simulink model "sim_finale_1"  (R2024a)
settings: Solver=FixedStepAuto  StartTime=0.0  StopTime=40  FixedStep=0.001  RelTol=1e-3
undefined symbols (not defined in the file): A_p, A_y, aero_variabile_con_M, Attitude_0, Attitude_riferimento, b, B_p, B_pz, B_y, B_yz, C_A, C_l, C_m_alpha, C_N_alpha, C_p, C_y, conv_cost_distE, conv_cost_distN, conv_cost_eta, conv_cost_p, conv_cost_y, conv_cost_zeta, D_pz, D_yz, Env, F, G_wE, G_wN, G_xp, G_xy, I_sp, inertia_p, inertia_s, inertia_tot, L, m_p, m_s, m_tot, MIL, Moderate, P_p, P_y, R, r_cp_cm, r_nozzle_cm, S_rif, spinta_variabile, T_c, T_r, v_0, V_r, VelocitB_riferimento, w_0
libraries: cstblocks x16, simulink_extras x5, slpidlib x4, simulink x3, aerolibasang x3, aerolibwind2 x3, matrix_library x2, shared6dof x2, aerolibatmos2 x2, aerolibutil x1, aerolibanim x1
(part 1 of 2)
settings Model: Creator=leo  LastModifiedBy=seraf

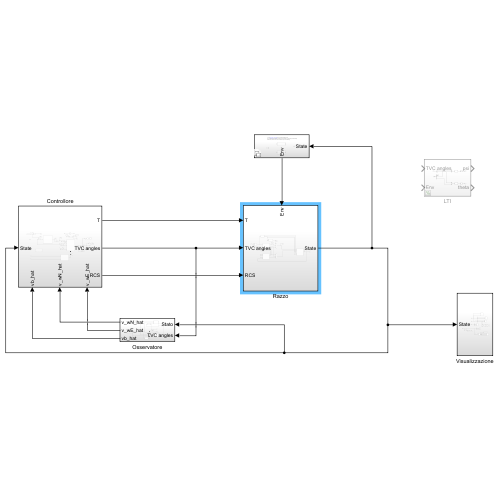
[thumbnail: Simulink's stored preview of the top-level diagram]
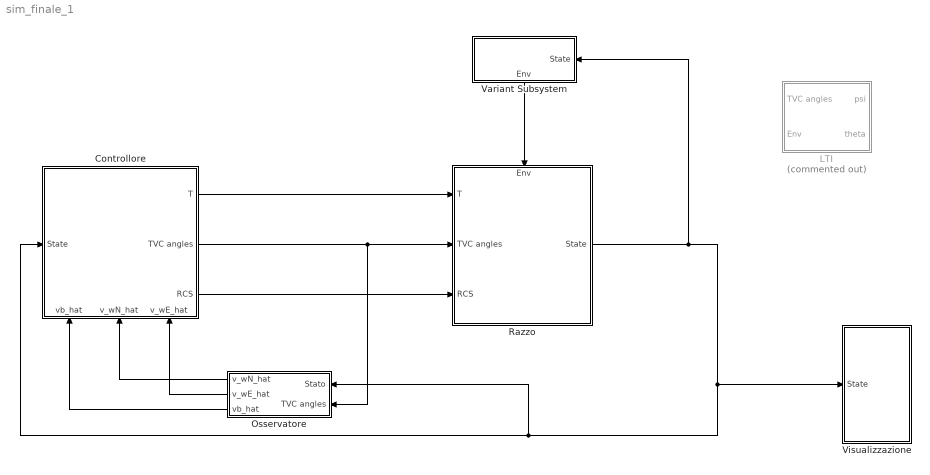
== system sim_finale_1 ==
  Controllore : Subsystem
      settings: PortSchema="{\"entries\":[{\"content\":{\"sides\":[{\"content\":{\"connectorIds\":[\"In1\"]},\"type\":\"ConnectorPlacement.EquallySpacedRectSide\",\"uuid\":\"b78b4143-dd7d-457a-9779-532a64936aad\"},{\"content\":{\"connectorIds\":[\"Out1\",\"Out2\",\"Out3\"],\"side\":\"RIGHT\"},\"type\":\"ConnectorPlacement.EquallySpacedRectSide\",\"uuid\":\"d89fe35f-6044-4244-8e7b-a164f9fa882f\"},{\"content\":{\"side\":\"TOP\"},\"type\":\"ConnectorPlacement.EquallySpacedRectSide\",\"uuid\":\"0b261906-0325-4b26-953a-0eb8d0997385\"},{\"content\":{\"connectorIds\":[\"In2\",\"In3\",\"In4\"],\"side\":\"BOTTOM\"},\"type\":\"ConnectorPlacement.EquallySpacedRectSide\",\"uuid\":\"57b86f82-ac2d-4b78-9198-4184c6b20db0\"}]},\"type\":\"ConnectorPlacement.EquallySpacedConnector\",\"uuid\":\"7c2dd957-a8a8-475b-8ed9-74adc6b1cefd\"}],\"packageUris\":[\"http://schema.mathworks.com/mf0/Connector/R2020b\"],\"version\":\"1.0\"}"
  LTI : Subsystem  Commented=on
  Osservatore : Subsystem
  Razzo : Subsystem
      settings: PortSchema="{\"entries\":[{\"content\":{\"sides\":[{\"content\":{\"connectorIds\":[\"In1\",\"In2\",\"In3\"]},\"type\":\"ConnectorPlacement.EquallySpacedRectSide\",\"uuid\":\"180f0abc-2401-4d87-8e99-f980c266d1e7\"},{\"content\":{\"connectorIds\":[\"Out1\"],\"side\":\"RIGHT\"},\"type\":\"ConnectorPlacement.EquallySpacedRectSide\",\"uuid\":\"394fd0a4-c6c4-4926-9ae8-64032c9821ed\"},{\"content\":{\"connectorIds\":[\"In4\"],\"side\":\"TOP\"},\"type\":\"ConnectorPlacement.EquallySpacedRectSide\",\"uuid\":\"a288fe65-10ee-4925-a534-5e3c09de9e1a\"}]},\"type\":\"ConnectorPlacement.EquallySpacedConnector\",\"uuid\":\"f348253f-31de-47bb-b686-6c6235580d40\"}],\"packageUris\":[\"http://schema.mathworks.com/mf0/Connector/R2020b\"],\"version\":\"1.0\"}"
  Variant Subsystem : Subsystem  Variant=on
      settings: PortSchema="{\"entries\":[{\"content\":{\"sides\":[{\"content\":{},\"type\":\"ConnectorPlacement.EquallySpacedRectSide\",\"uuid\":\"da193b29-da6f-4442-8838-85822d0fc2da\"},{\"content\":{\"connectorIds\":[\"In1\"],\"side\":\"RIGHT\"},\"type\":\"ConnectorPlacement.EquallySpacedRectSide\",\"uuid\":\"175a63c7-dae9-42af-bcb0-1cf5a0daaa56\"},{\"content\":{\"side\":\"TOP\"},\"type\":\"ConnectorPlacement.EquallySpacedRectSide\",\"uuid\":\"021eae39-a2a3-4258-8f48-6aaa3d6bb465\"},{\"content\":{\"connectorIds\":[\"Out1\"],\"side\":\"BOTTOM\"},\"type\":\"ConnectorPlacement.EquallySpacedRectSide\",\"uuid\":\"d77f05be-424c-4b1f-8c52-f4d487af08f8\"}]},\"type\":\"ConnectorPlacement.EquallySpacedConnector\",\"uuid\":\"9e6b8849-3b74-4285-b295-863aaca4edda\"}],\"packageUris\":[\"http://schema.mathworks.com/mf0/Connector/R2020b\"],\"version\":\"1.0\"}"
  Visualizzazione : Subsystem
  wires:
  Controllore/1(T) -> Razzo/1(T)
  Controllore/2(TVC angles) -> Razzo/2(TVC angles), Osservatore/2(TVC angles)
  Controllore/3(RCS) -> Razzo/3(RCS)
  Osservatore/1(v_wN_hat) -> Controllore/3(v_wN_hat)
  Osservatore/2(v_wE_hat) -> Controllore/4(v_wE_hat)
  Razzo/1(State) -> Variant Subsystem/1(State), Controllore/1(State), Osservatore/1(Stato), Visualizzazione/1(State)
  Osservatore/3(vb_hat) -> Controllore/2(vb_hat)
  Variant Subsystem/1(Env) -> Razzo/4(Env)

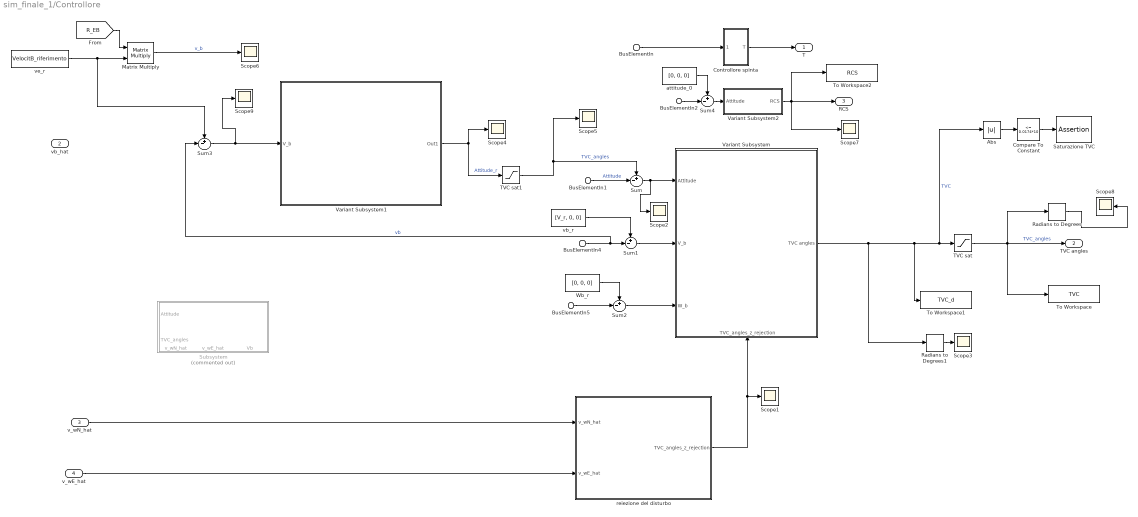
== system sim_finale_1/Controllore ==
  BusElementIn : Inport  PortName=State  Element=Ve
  BusElementIn5 : Inport  PortName=State  Element=Wb
  BusElementIn1 : Inport  PortName=State  Element=Attitude
  BusElementIn2 : Inport  PortName=State  Element=Attitude
  BusElementIn4 : Inport  PortName=State  Element=Vb
  vb_hat : Inport  Port=2
  v_wN_hat : Inport  Port=3
  v_wE_hat : Inport  Port=4
  Abs : Abs  SaturateOnIntegerOverflow=off
  Compare To Constant : simulink/Logic and Bit Operations/Compare To Constant  relop=<=  const=0.0174*10  OutDataTypeStr=boolean
  Controllore spinta : Subsystem
  Matrix Multiply : Product  Multiplication=Matrix(*)
  Radians to Degrees : simulink_extras/Transformations/Radians to Degrees
  Radians to Degrees1 : simulink_extras/Transformations/Radians to Degrees
  Saturazione TVC : Assertion  AssertionFailFcn="disp(\"sat TVC\");"  StopWhenAssertionFail=off
  Scope{1..9} (9 alike) : Scope
  Subsystem : Subsystem  Commented=on
      settings: PortSchema="{\"entries\":[{\"content\":{\"sides\":[{\"content\":{\"connectorIds\":[\"In1\",\"In2\"]},\"type\":\"ConnectorPlacement.EquallySpacedRectSide\",\"uuid\":\"7d03ec52-65f5-4749-86a5-4e4c2783c638\"},{\"content\":{\"side\":\"RIGHT\"},\"type\":\"ConnectorPlacement.EquallySpacedRectSide\",\"uuid\":\"e1268fd9-4d44-4554-a2b2-3dcef73677eb\"},{\"content\":{\"side\":\"TOP\"},\"type\":\"ConnectorPlacement.EquallySpacedRectSide\",\"uuid\":\"d645f998-d977-4111-8b81-622ab61ecf1a\"},{\"content\":{\"connectorIds\":[\"In3\",\"In4\",\"Out1\"],\"side\":\"BOTTOM\"},\"type\":\"ConnectorPlacement.EquallySpacedRectSide\",\"uuid\":\"b191ee85-0885-4cad-8a49-973173d49373\"}]},\"type\":\"ConnectorPlacement.EquallySpacedConnector\",\"uuid\":\"8035aa71-bfb6-4343-86e2-3a1cc86d2cc7\"}],\"packageUris\":[\"http://schema.mathworks.com/mf0/Connector/R2020b\"],\"version\":\"1.0\"}"
  Sum{,1..4} (5 alike) : Sum  Inputs=+-|
  TVC sat : Saturate  UpperLimit=0.0174*10  LowerLimit=-0.0174*10
  TVC sat1 : Saturate  UpperLimit=0.085  LowerLimit=-0.085
  To Workspace : ToWorkspace  VariableName=TVC  SaveFormat=Timeseries  SampleTime=-1
  To Workspace1 : ToWorkspace  VariableName=TVC_d  SaveFormat=Timeseries  SampleTime=-1
  To Workspace2 : ToWorkspace  VariableName=RCS  SaveFormat=Timeseries  SampleTime=-1
  Variant Subsystem : Subsystem  Variant=on
      settings: PortSchema="{\"entries\":[{\"content\":{\"sides\":[{\"content\":{\"connectorIds\":[\"In1\",\"In2\",\"In3\"]},\"type\":\"ConnectorPlacement.EquallySpacedRectSide\",\"uuid\":\"66b0b15b-ed6b-4b76-89bf-2c64339f4943\"},{\"content\":{\"connectorIds\":[\"Out1\"],\"side\":\"RIGHT\"},\"type\":\"ConnectorPlacement.EquallySpacedRectSide\",\"uuid\":\"d7e4ce79-fa2c-4df2-bf14-20d4b93c516e\"},{\"content\":{\"side\":\"TOP\"},\"type\":\"ConnectorPlacement.EquallySpacedRectSide\",\"uuid\":\"6c4a5895-245f-4b03-9ae1-4531346de6c9\"},{\"content\":{\"connectorIds\":[\"In4\"],\"side\":\"BOTTOM\"},\"type\":\"ConnectorPlacement.EquallySpacedRectSide\",\"uuid\":\"f799af13-07e4-4630-a5d1-2cd1e27b70f0\"}]},\"type\":\"ConnectorPlacement.EquallySpacedConnector\",\"uuid\":\"81d951f5-5656-48a6-8dfe-886e27de443b\"}],\"packageUris\":[\"http://schema.mathworks.com/mf0/Connector/R2020b\"],\"version\":\"1.0\"}"
  Variant Subsystem1 : Subsystem  Variant=on
  Variant Subsystem2 : Subsystem  Variant=on
  Wb_r : Constant  Value=[0, 0, 0]
  attitude_0 : Constant  Value=[0, 0, 0]
  reiezione del disturbo : Subsystem  Variant=on
  vb_r : Constant  Value=[V_r, 0, 0]
  ve_r : Constant  Value=VelocitB_riferimento
  T : Outport
  TVC angles : Outport  Port=2
  RCS : Outport  Port=3
  wires:
  BusElementIn/1 -> Controllore spinta/1(State)
  Controllore spinta/1(T) -> T/1
  BusElementIn2/1 -> Sum4/2
  Radians to Degrees/1 -> Scope8/1
  BusElementIn1/1 -> Sum/2  "Attitude"
  Sum/1 -> Scope2/1, Variant Subsystem/1(Attitude)
  Sum1/1 -> Variant Subsystem/2(V_b)
  vb_r/1 -> Sum1/1
  Wb_r/1 -> Sum2/1
  BusElementIn5/1 -> Sum2/2
  Sum2/1 -> Variant Subsystem/3(W_b)
  Variant Subsystem/1(TVC angles) -> Radians to Degrees1/1, To Workspace1/1, Abs/1, TVC sat/1  "TVC"
  v_wE_hat/1 -> reiezione del disturbo/2(v_wE_hat)
  v_wN_hat/1 -> reiezione del disturbo/1(v_wN_hat)
  reiezione del disturbo/1(TVC_angles_z_rejection) -> Scope1/1, Variant Subsystem/4(TVC_angles_z_rejection)
  TVC sat/1 -> TVC angles/1, To Workspace/1, Radians to Degrees/1  "TVC_angles"
  Compare To Constant/1 -> Saturazione TVC/1
  Abs/1 -> Compare To Constant/1
  Radians to Degrees1/1 -> Scope3/1
  Variant Subsystem1/1(Out1) -> TVC sat1/1, Scope4/1  "Attitude_r"
  Sum3/1 -> Scope9/1, Variant Subsystem1/1(V_b)
  BusElementIn4/1 -> Sum3/2, Sum1/2  "vb"
  Matrix Multiply/1 -> Scope6/1  "v_b"
  ve_r/1 -> Sum3/1, Matrix Multiply/2
  [R_EB] -> Matrix Multiply/1
  TVC sat1/1 -> Scope5/1, Sum/1  "TVC_angles"
  Sum4/1 -> Variant Subsystem2/1(Attitude)
  attitude_0/1 -> Sum4/1
  Variant Subsystem2/1(RCS) -> To Workspace2/1, RCS/1, Scope7/1

== system sim_finale_1/LTI ==
  TVC angles : Inport
  BusElementIn : Inport  Port=2  PortName=Env  Element=WindVelocity
  Demux : Demux  Outputs=3
  Demux1 : Demux  Outputs=2
  LTI Pitch : StateSpace  A=A_p  B=B_pz  C=C_p  D=D_pz  InitialCondition=[v_0(3); w_0(2); Attitude_0(2)]
  LTI Yaw : StateSpace  A=A_y  B=B_yz  C=C_y  D=D_yz  InitialCondition=[v_0(2); w_0(3); Attitude_0(3)]
  Mux : Mux  Inputs=2
  Mux1 : Mux  Inputs=2
  Radians to Degrees : simulink_extras/Transformations/Radians to Degrees
  Radians to Degrees1 : simulink_extras/Transformations/Radians to Degrees
  Terminator : Terminator
  psi : Outport
  theta : Outport  Port=2
  wires:
  Demux/2 -> Mux1/2  "v_wN"
  LTI Pitch/1 -> Radians to Degrees1/1
  Demux1/1 -> Mux1/1  "zeta"
  Mux1/1 -> LTI Yaw/1
  Mux/1 -> LTI Pitch/1
  LTI Yaw/1 -> Radians to Degrees/1  "psi"
  BusElementIn/1 -> Demux/1
  Demux/1 -> Terminator/1
  Demux/3 -> Mux/2  "v_wE"
  TVC angles/1 -> Demux1/1
  Demux1/2 -> Mux/1  "eta"
  Radians to Degrees/1 -> psi/1
  Radians to Degrees1/1 -> theta/1

== system sim_finale_1/Osservatore ==
  BusElementIn : Inport  PortName=Stato  Element=Attitude
  BusElementIn1 : Inport  PortName=Stato  Element=Vb
  BusElementIn2 : Inport  PortName=Stato  Element=Wb
  TVC angles : Inport  Port=2
  Demux : Demux  Outputs=2
  Ground : Ground
  Mux : Mux  Inputs=3
  PITCH : Subsystem
  Scope : Scope  NumInputPorts=2
  Scope1 : Scope
  Subsystem : Subsystem
  Subsystem1 : Subsystem
  Subsystem2 : Subsystem
  YAW : Subsystem
  v_wN_hat : Outport
  v_wE_hat : Outport  Port=2
  vb_hat : Outport  Port=3
  wires:
  TVC angles/1 -> Demux/1
  BusElementIn/1 -> Subsystem2/1(In1)
  BusElementIn1/1 -> Subsystem2/2(In2)
  BusElementIn2/1 -> Subsystem2/3(In3)
  Demux/1 -> YAW/2(zeta)  "zeta"
  Demux/2 -> PITCH/2(eta)  "eta"
  Subsystem2/1(x_yaw) -> YAW/1(x_y)
  Subsystem2/2(x_pitch) -> PITCH/1(x_p)
  Subsystem1/1(v_wN_hat) -> v_wN_hat/1, Scope/1, YAW/3(v_wN_hat)
  Subsystem/1(v_wE_hat) -> PITCH/3(v_wE_hat), v_wE_hat/1, Scope/2
  PITCH/1(e_p) -> Subsystem/1(e_p)
  YAW/1(e_y) -> Subsystem1/1(e_y), Scope1/1
  YAW/2(v) -> Mux/2
  PITCH/2(w) -> Mux/3
  Ground/1 -> Mux/1
  Mux/1 -> vb_hat/1

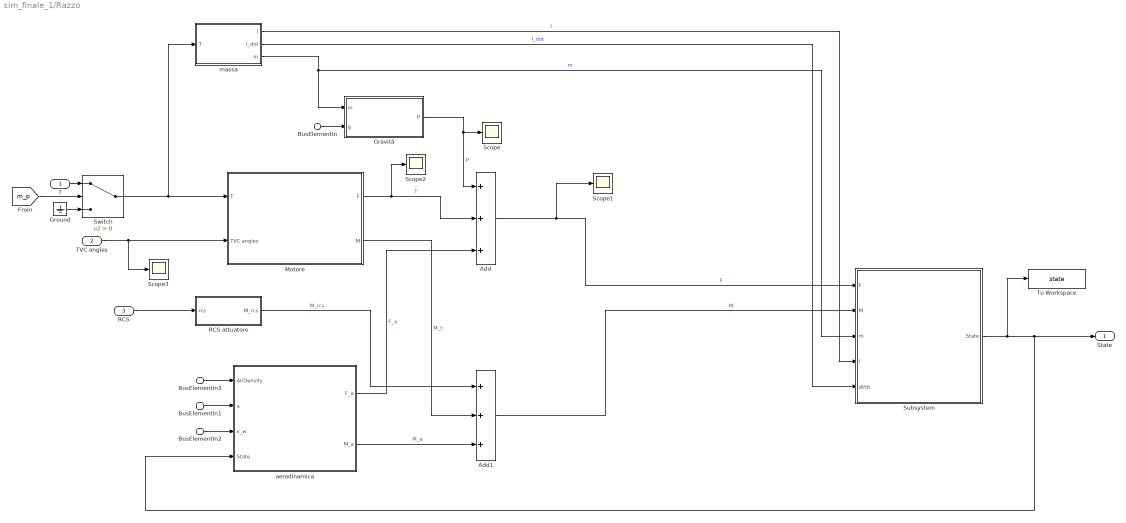
== system sim_finale_1/Razzo ==
  T : Inport
  TVC angles : Inport  Port=2
  RCS : Inport  Port=3
  BusElementIn2 : Inport  Port=4  PortName=Env  Element=Wind
  BusElementIn : Inport  Port=4  PortName=Env  Element=Gravity
  BusElementIn1 : Inport  Port=4  PortName=Env  Element=SpeedOfSound
  BusElementIn3 : Inport  Port=4  PortName=Env  Element=AirDensity
  Add : Sum  Inputs=+++
  Add1 : Sum  Inputs=+++
  Gravità : Subsystem
  Ground : Ground
  Motore : Subsystem
  RCS attuatore : Subsystem
  Scope{,1..3} (4 alike) : Scope
  Subsystem : Subsystem
  Switch : Switch  Criteria=u2 > Threshold  SaturateOnIntegerOverflow=off  InputSameDT=off
  To Workspace : ToWorkspace  VariableName=state  SaveFormat=Timeseries  SampleTime=-1
  aerodinamica : Subsystem
  massa : Subsystem  Variant=on  VariantControl=Subsystem1
  State : Outport
  wires:
  BusElementIn2/1 -> aerodinamica/3(v_w)
  BusElementIn3/1 -> aerodinamica/1(AirDensity)
  Motore/1(F) -> Scope2/1, Add/2  "T"
  aerodinamica/2(M_a) -> Add1/3  "M_a"
  aerodinamica/1(F_a) -> Add/3  "F_a"
  Motore/2(M) -> Add1/2  "M_t"
  Switch/1 -> massa/1(T), Motore/1(T)
  TVC angles/1 -> Scope3/1, Motore/2(TVC angles)
  BusElementIn1/1 -> aerodinamica/2(" a")
  massa/2(I_dot) -> Subsystem/5(dI/dt)  "I_dot"
  massa/3(m) -> Gravità/1(m), Subsystem/3(m)  "m"
  Gravità/1(P) -> Scope/1, Add/1  "P"
  Ground/1 -> Switch/3
  T/1 -> Switch/1
  massa/1(I) -> Subsystem/4(I)  "I"
  Subsystem/1(State) -> To Workspace/1, State/1, aerodinamica/4(State)
  Add/1 -> Scope1/1, Subsystem/1(F)  "F"
  [m_p] -> Switch/2
  RCS/1 -> RCS attuatore/1(rcs)
  RCS attuatore/1(M_rcs) -> Add1/1  "M_rcs"
  Add1/1 -> Subsystem/2(M)  "M"
  BusElementIn/1 -> Gravità/2(g)

== system sim_finale_1/Variant Subsystem ==
  note: 1) Add Subsystem or Model blocks as valid variant choices.
      | 2) You cannot connect blocks at this level. At simulation, connectivity is automatically
      | determined, based on the active variant and port name matching.
  State : Inport
  meno reale : Subsystem  VariantControl=tutto_realistico==0
  reale : Subsystem  VariantControl=tutto_realistico==1
  Env : Outport

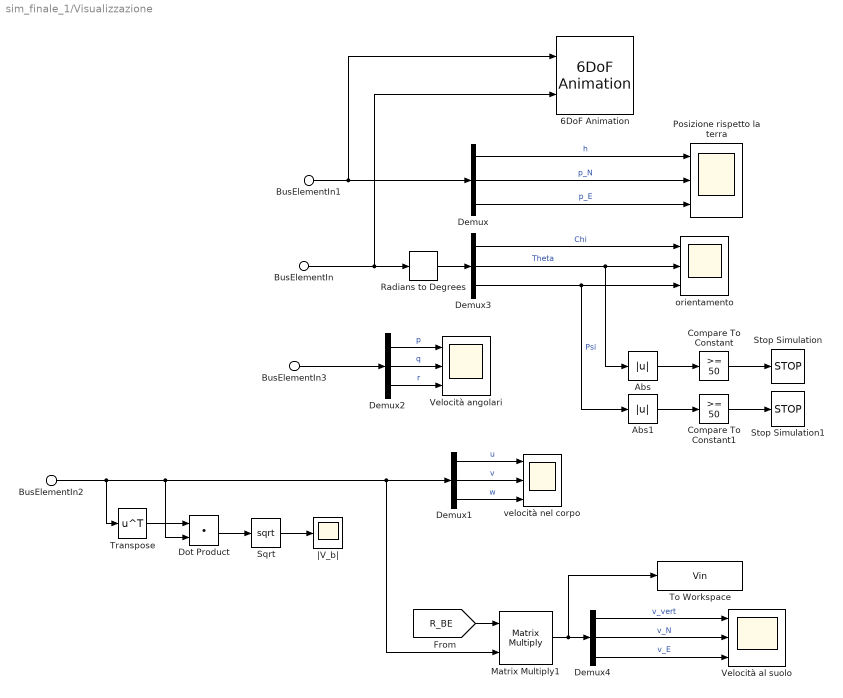
== system sim_finale_1/Visualizzazione ==
  BusElementIn : Inport  PortName=State  Element=Attitude
  BusElementIn1 : Inport  PortName=State  Element=Xe
  BusElementIn2 : Inport  PortName=State  Element=Vb
  BusElementIn3 : Inport  PortName=State  Element=Wb
  6DoF Animation : aerolibanim/6DoF Animation  u1=[0 4000 -2000 2000 -5000 -3000]  u2=0.05  u3=10  u4=[10 0 0]  u5=Fly alongside  u6=[0 500 0]  u7=15  u8=off
  Abs : Abs  SaturateOnIntegerOverflow=off
  Abs1 : Abs  SaturateOnIntegerOverflow=off
  Compare To Constant : simulink/Logic and Bit Operations/Compare To Constant  relop=>=  const=50  OutDataTypeStr=boolean
  Compare To Constant1 : simulink/Logic and Bit Operations/Compare To Constant  relop=>=  const=50  OutDataTypeStr=boolean
  Demux{,1..4} (5 alike) : Demux  Outputs=3
  Dot Product : DotProduct  OutDataTypeStr=Inherit: Inherit via internal rule
  Matrix Multiply1 : Product  Multiplication=Matrix(*)
  Posizione rispetto la terra : Scope  NumInputPorts=3
  Radians to Degrees : simulink_extras/Transformations/Radians to Degrees
  Sqrt : Sqrt
  Stop Simulation : Stop
  Stop Simulation1 : Stop
  To Workspace : ToWorkspace  VariableName=Vin  SaveFormat=Timeseries  SampleTime=-1
  Transpose : Math  Operator=transpose
  Velocità al suolo : Scope  NumInputPorts=3
  Velocità angolari : Scope  NumInputPorts=3
  orientamento : Scope  NumInputPorts=3
  velocità nel corpo : Scope  NumInputPorts=3
  |V_b| : Scope
  wires:
  BusElementIn2/1 -> Matrix Multiply1/2, Demux1/1, Dot Product/2, Transpose/1
  Matrix Multiply1/1 -> To Workspace/1, Demux4/1
  Demux/3 -> Posizione rispetto la terra/3  "p_E"
  Demux4/1 -> Velocità al suolo/1  "v_vert"
  Demux1/2 -> velocità nel corpo/2  "v"
  Demux/1 -> Posizione rispetto la terra/1  "h"
  [R_BE] -> Matrix Multiply1/1
  Demux4/3 -> Velocità al suolo/3  "v_E"
  Demux1/1 -> velocità nel corpo/1  "u"
  Demux4/2 -> Velocità al suolo/2  "v_N"
  Demux1/3 -> velocità nel corpo/3  "w"
  Demux/2 -> Posizione rispetto la terra/2  "p_N"
  BusElementIn1/1 -> 6DoF Animation/1, Demux/1
  BusElementIn/1 -> Radians to Degrees/1, 6DoF Animation/2
  Demux3/1 -> orientamento/1  "Chi"
  Demux3/2 -> Abs/1, orientamento/2  "Theta"
  Demux3/3 -> Abs1/1, orientamento/3  "Psi"
  BusElementIn3/1 -> Demux2/1
  Demux2/1 -> Velocità angolari/1  "p"
  Demux2/2 -> Velocità angolari/2  "q"
  Demux2/3 -> Velocità angolari/3  "r"
  Radians to Degrees/1 -> Demux3/1
  Transpose/1 -> Dot Product/1
  Dot Product/1 -> Sqrt/1
  Sqrt/1 -> |V_b|/1
  Compare To Constant/1 -> Stop Simulation/1
  Compare To Constant1/1 -> Stop Simulation1/1
  Abs/1 -> Compare To Constant/1
  Abs1/1 -> Compare To Constant1/1

== system sim_finale_1/Controllore/Controllore spinta ==
  State : Inport
  Constant : Constant  Value=T_c
  Constant1 : Constant  Value=T_r
  Constant2 : Constant  Value=spinta_variabile
  Constant3 : Constant  Value=V_r
  Demux : Demux  Outputs=3
  Ground : Ground
  PID Controller : slpidlib/PID Controller  Controller=PID  Form=Parallel  TimeDomain=Continuous-time  UseExternalTs=off  SampleTime=-1  IntegratorMethod=Forward Euler  FilterMethod=Forward Euler  ControllerParametersSource=internal  P=-285376.920173574  I=-25448.2811589102  UseKiTs=off  D=7697.0953395777  UseExternalDerivativeSource=off  N=37.0759237846768  UseFilter=on  TunerSelectOption=Transfer Function Based (PID Tuner App)  InitialConditionSource=internal  InitialConditionForIntegrator=0  InitialConditionForFilter=0  DifferentiatorICPrevScaledInput=0  ExternalReset=none  TrackingMode=off  Kt=1  LimitOutput=off  SatLimitsSource=internal  UpperSaturationLimit=inf  LowerSaturationLimit=-inf  LinearizeAsGain=on  AntiWindupMode=none  Kb=1  LimitIntegrator=off  UpperIntegratorSaturationLimit=inf  LowerIntegratorSaturationLimit=-inf  POutMin=[]  POutMax=[]  IOutMin=[]  IOutMax=[]  DOutMin=[]  DOutMax=[]  NOutMin=[]  NOutMax=[]  SumOutMin=[]  SumOutMax=[]  SaturationOutMin=[]  SaturationOutMax=[]  PParamMin=[]  PParamMax=[]  IParamMin=[]  IParamMax=[]  DParamMin=[]  DParamMax=[]  NParamMin=[]  NParamMax=[]  KbParamMin=[]  KbParamMax=[]  KtParamMin=[]  KtParamMax=[]  KbOutMin=[]  KbOutMax=[]  KtOutMin=[]  KtOutMax=[]  IntegratorOutMin=[]  IntegratorOutMax=[]  FilterOutMin=[]  FilterOutMax=[]  SumI1OutMin=[]  SumI1OutMax=[]  SumI2OutMin=[]  SumI2OutMax=[]  SumI3OutMin=[]  SumI3OutMax=[]  SumI4OutMin=[]  SumI4OutMax=[]  SumDOutMin=[]  SumDOutMax=[]  DifferentiatorOutMin=[]  DifferentiatorOutMax=[]  FilterDiffOutCoefMin=[]  FilterDiffOutCoefMax=[]  ReciprocalOutMin=[]  ReciprocalOutMax=[]  SumDenOutMin=[]  SumDenOutMax=[]  SumNumOutMin=[]  SumNumOutMax=[]  DivideOutMin=[]  DivideOutMax=[]  UdiffTsProdOutMin=[]  UdiffTsProdOutMax=[]  NTsProdOutMin=[]  NTsProdOutMax=[]  UintegralTsProdOutMin=[]  UintegralTsProdOutMax=[]  UngainTsProdOutMin=[]  UngainTsProdOutMax=[]  ClampingZeroOutDataTypeStr=Inherit: Inherit via back propagation  ClampingZeroOutMin=[]  ClampingZeroOutMax=[]  FilterDenConstantOutDataTypeStr=Inherit: Inherit via back propagation  FilterDenConstantOutMin=[]  FilterDenConstantOutMax=[]  PCopyOutDataTypeStr=Inherit: Inherit via back propagation  PCopyOutMin=[]  PCopyOutMax=[]  NCopyOutDataTypeStr=Inherit: Inherit via back propagation  NCopyOutMin=[]  NCopyOutMax=[]  IntegratorContinuousStateAttributes=''  IntegratorStateMustResolveToSignalObject=off  IntegratorRTWStateStorageClass=Auto  FilterContinuousStateAttributes=''  FilterStateMustResolveToSignalObject=off  FilterRTWStateStorageClass=Auto  ParallelPVariant=InternalParameters  IdealPVariant=Disabled  IVariant=InternalParameters  DVariant=InternalParameters  IntegratorVariant=Continuous  SatVariant=Disabled  AWVariant=Passthrough  PCopyVariant=Disabled  TRVariant=Disabled  FdbkBlocksVariant=Forward  IdealPFdbkVariant=Disabled  SatFdbkVariant=Disabled  DerivativeFilterVariant=ContFilter  NVariant=InternalParameters  NCopyVariant=Disabled  FilterICVariant=InternalICsFilter  IntegratorICVariant=InternalICs  ExternalResetVariant=Disabled  TRSumVariant=Passthrough  SumFdbkVariant=Disabled  SumVariant=Sum_PID  TsampFilterVariant=InternalTs  TsampNgainVariant=Passthrough  TsampIntegralVariant=Disabled_SignalSpec  ExternalSaturationOutDataTypeStr=Inherit: Same as second input  DerivativeSourceVariant=ErrorSignal
  Scope : Scope
  Sum : Sum  Inputs=|+-
  Sum1 : Sum  Inputs=++|
  Switch : Switch  Criteria=u2 > Threshold  SaturateOnIntegerOverflow=off  InputSameDT=off
  Terminator : Terminator
  Terminator1 : Terminator
  Terminator2 : Terminator
  T : Outport
  wires:
  PID Controller/1 -> Terminator2/1
  State/1 -> Demux/1
  Demux/3 -> Terminator1/1
  Constant3/1 -> Sum/2
  Ground/1 -> Sum1/2
  Sum1/1 -> T/1, Scope/1
  Sum/1 -> PID Controller/1
  Demux/1 -> Sum/1  "u"
  Demux/2 -> Terminator/1
  Constant/1 -> Switch/1
  Switch/1 -> Sum1/1
  Constant1/1 -> Switch/3
  Constant2/1 -> Switch/2

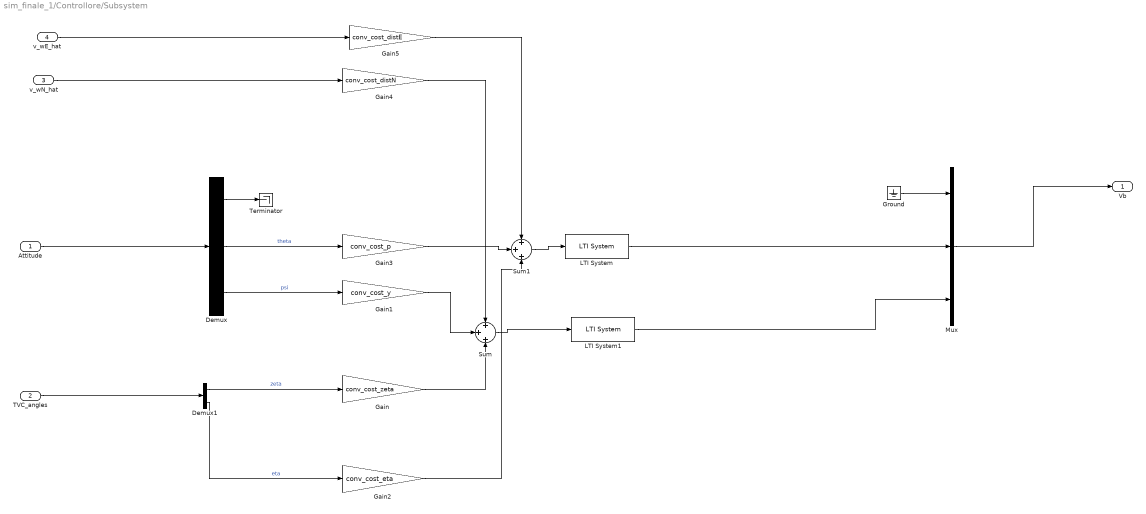
== system sim_finale_1/Controllore/Subsystem ==
  Attitude : Inport
  TVC_angles : Inport  Port=2
  v_wN_hat : Inport  Port=3
  v_wE_hat : Inport  Port=4
  Demux : Demux  Outputs=3
  Demux1 : Demux  Outputs=2
  Gain : Gain  Gain=conv_cost_zeta
  Gain1 : Gain  Gain=conv_cost_y
  Gain2 : Gain  Gain=conv_cost_eta
  Gain3 : Gain  Gain=conv_cost_p
  Gain4 : Gain  Gain=conv_cost_distN
  Gain5 : Gain  Gain=conv_cost_distE
  Ground : Ground
  LTI System : cstblocks/LTI System  sys=conv_den_p  IC=[]  PadeOrder=0
  LTI System1 : cstblocks/LTI System  sys=conv_den_y  IC=[]  PadeOrder=0
  Mux : Mux  Inputs=3
  Sum : Sum  Inputs=+|+|+
  Sum1 : Sum  Inputs=+|+|+
  Terminator : Terminator
  Vb : Outport
  wires:
  Attitude/1 -> Demux/1
  Demux/2 -> Gain3/1  "theta"
  Demux/3 -> Gain1/1  "psi"
  Mux/1 -> Vb/1
  LTI System1/1 -> Mux/3
  Demux/1 -> Terminator/1
  Ground/1 -> Mux/1
  TVC_angles/1 -> Demux1/1
  Demux1/1 -> Gain/1  "zeta"
  Sum/1 -> LTI System1/1
  Demux1/2 -> Gain2/1  "eta"
  Sum1/1 -> LTI System/1
  LTI System/1 -> Mux/2
  Gain3/1 -> Sum1/2
  Gain2/1 -> Sum1/3
  v_wN_hat/1 -> Gain4/1
  v_wE_hat/1 -> Gain5/1
  Gain/1 -> Sum/3
  Gain1/1 -> Sum/2
  Gain4/1 -> Sum/1
  Gain5/1 -> Sum1/1

== system sim_finale_1/Controllore/Variant Subsystem ==
  Attitude : Inport
  V_b : Inport  Port=2
  W_b : Inport  Port=3
  TVC_angles_z_rejection : Inport  Port=4
  "Controllore 2: rlocus sforzo di TVC minore " : Subsystem  VariantControl=tipo_controllo==6
  PID : Subsystem  VariantControl=tipo_controllo==1
  tune : Subsystem  VariantControl=tipo_controllo==0
  TVC angles : Outport

== system sim_finale_1/Controllore/Variant Subsystem1 ==
  note: 1) Add Subsystem or Model blocks as valid variant choices.
      | 2) You cannot connect blocks at this level. At simulation, connectivity is automatically
      | determined, based on the active variant and port name matching.
  V_b : Inport
  No controllore velocità : Subsystem  VariantControl=controllo_velcit==0
  PID : Subsystem  VariantControl=controllo_velcit==1
  Out1 : Outport

== system sim_finale_1/Controllore/Variant Subsystem2 ==
  Attitude : Inport
  mio controllo : Subsystem  VariantControl=controllo_roll==1
  sbagliato : Subsystem  VariantControl=controllo_roll==-1
  tune : Subsystem  VariantControl=(default)
  RCS : Outport

== system sim_finale_1/Controllore/reiezione del disturbo ==
  v_wN_hat : Inport
  v_wE_hat : Inport  Port=2
  Vuoto : Subsystem  VariantControl=(default)
  frequenza controllore 3 : Subsystem  VariantControl=tipo_controllo==3
  frequenza controllore 4 : Subsystem  VariantControl=tipo_controllo==4
  frequenza controllore 7 : Subsystem  VariantControl=tipo_controllo==7
  TVC_angles_z_rejection : Outport

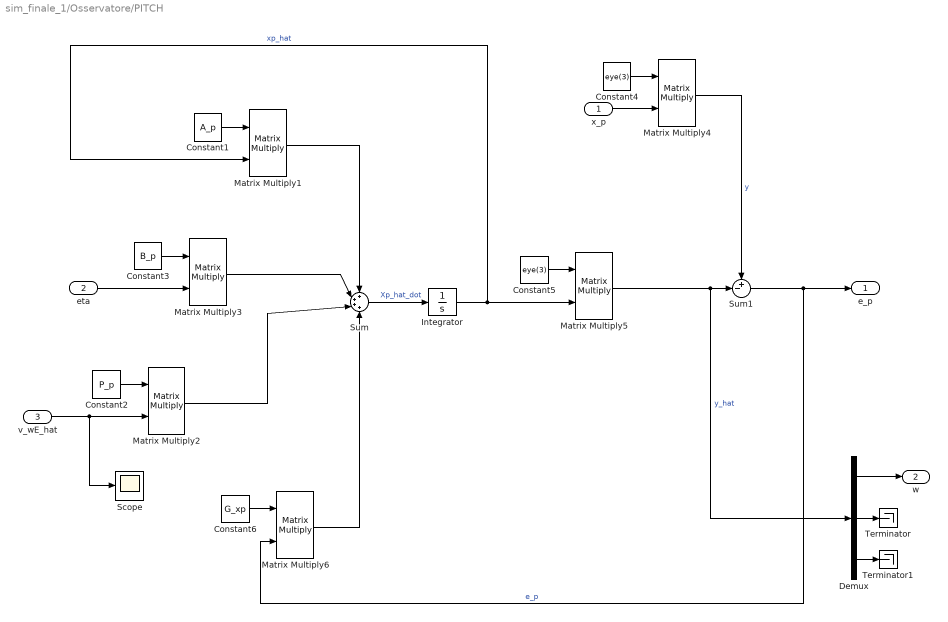
== system sim_finale_1/Osservatore/PITCH ==
  x_p : Inport
  eta : Inport  Port=2
  v_wE_hat : Inport  Port=3
  Constant1 : Constant  Value=A_p  VectorParams1D=off
  Constant2 : Constant  Value=P_p  VectorParams1D=off
  Constant3 : Constant  Value=B_p  VectorParams1D=off
  Constant4 : Constant  Value=eye(3)  VectorParams1D=off
  Constant5 : Constant  Value=eye(3)  VectorParams1D=off
  Constant6 : Constant  Value=G_xp  VectorParams1D=off
  Demux : Demux  Outputs=3
  Integrator : Integrator
  Matrix Multiply{1..6} (6 alike) : Product  Multiplication=Matrix(*)
  Scope : Scope
  Sum : Sum  Inputs=++++
  Sum1 : Sum  Inputs=+-|
  Terminator : Terminator
  Terminator1 : Terminator
  e_p : Outport
  w : Outport  Port=2
  wires:
  v_wE_hat/1 -> Scope/1, Matrix Multiply2/2
  Constant5/1 -> Matrix Multiply5/1
  Integrator/1 -> Matrix Multiply5/2, Matrix Multiply1/2  "xp_hat"
  eta/1 -> Matrix Multiply3/2
  Constant1/1 -> Matrix Multiply1/1
  Matrix Multiply4/1 -> Sum1/1  "y"
  Constant2/1 -> Matrix Multiply2/1
  Matrix Multiply6/1 -> Sum/4
  Matrix Multiply3/1 -> Sum/2
  Constant3/1 -> Matrix Multiply3/1
  x_p/1 -> Matrix Multiply4/2
  Sum1/1 -> Matrix Multiply6/2, e_p/1  "e_p"
  Sum/1 -> Integrator/1  "Xp_hat_dot"
  Constant6/1 -> Matrix Multiply6/1
  Matrix Multiply1/1 -> Sum/1
  Matrix Multiply2/1 -> Sum/3
  Constant4/1 -> Matrix Multiply4/1
  Demux/1 -> w/1
  Matrix Multiply5/1 -> Demux/1, Sum1/2  "y_hat"
  Demux/3 -> Terminator1/1
  Demux/2 -> Terminator/1

== system sim_finale_1/Osservatore/Subsystem ==
  e_p : Inport
  Constant : Constant  Value=G_wE  VectorParams1D=off
  Integrator : Integrator
  Matrix Multiply : Product  Multiplication=Matrix(*)
  v_wE_hat : Outport
  wires:
  Integrator/1 -> v_wE_hat/1
  Constant/1 -> Matrix Multiply/1
  Matrix Multiply/1 -> Integrator/1
  e_p/1 -> Matrix Multiply/2

== system sim_finale_1/Osservatore/Subsystem1 ==
  e_y : Inport
  Constant1 : Constant  Value=G_wN  VectorParams1D=off
  Integrator : Integrator
  Matrix Multiply : Product  Multiplication=Matrix(*)
  v_wN_hat : Outport
  wires:
  Constant1/1 -> Matrix Multiply/1
  e_y/1 -> Matrix Multiply/2
  Integrator/1 -> v_wN_hat/1
  Matrix Multiply/1 -> Integrator/1

== system sim_finale_1/Osservatore/Subsystem2 ==
  In1 : Inport
  In2 : Inport  Port=2
  In3 : Inport  Port=3
  Demux1 : Demux  Outputs=3
  Demux2 : Demux  Outputs=3
  Demux3 : Demux  Outputs=3
  Mux : Mux  Inputs=3
  Mux2 : Mux  Inputs=3
  Terminator : Terminator
  Terminator1 : Terminator
  Terminator2 : Terminator
  x_yaw : Outport
  x_pitch : Outport  Port=2
  wires:
  In2/1 -> Demux2/1
  Mux2/1 -> x_pitch/1  "x_pitch"
  Mux/1 -> x_yaw/1  "x_yaw"
  Demux1/3 -> Mux/3  "psi"
  Demux3/1 -> Terminator2/1
  Demux2/3 -> Mux2/1  "w"
  Demux3/3 -> Mux/2  "r"
  Demux3/2 -> Mux2/2  "q"
  In3/1 -> Demux3/1
  Demux2/1 -> Terminator1/1
  Demux1/2 -> Mux2/3  "theta"
  Demux2/2 -> Mux/1  "v"
  In1/1 -> Demux1/1
  Demux1/1 -> Terminator/1

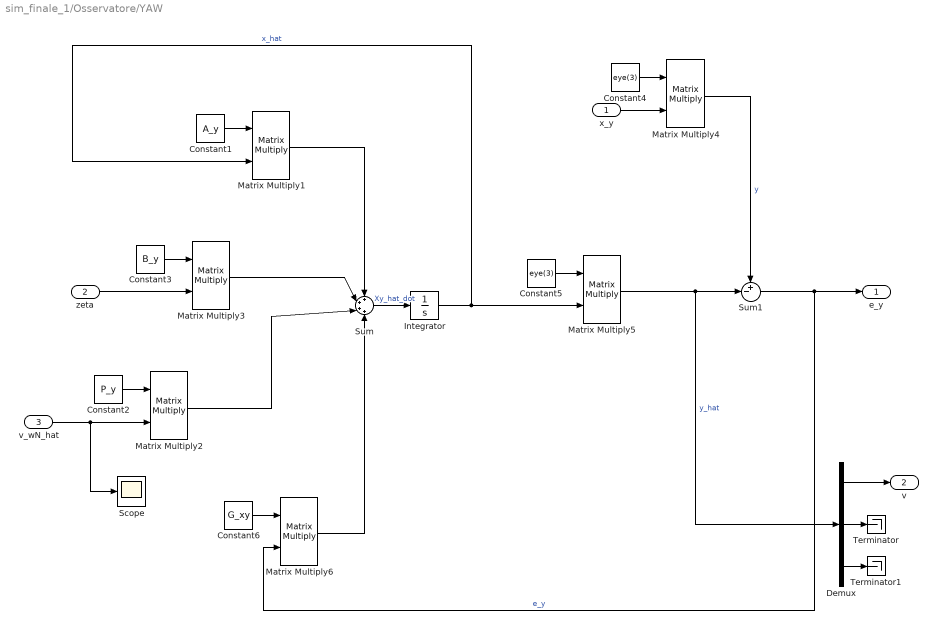
== system sim_finale_1/Osservatore/YAW ==
  x_y : Inport
  zeta : Inport  Port=2
  v_wN_hat : Inport  Port=3
  Constant1 : Constant  Value=A_y  VectorParams1D=off
  Constant2 : Constant  Value=P_y  VectorParams1D=off
  Constant3 : Constant  Value=B_y  VectorParams1D=off
  Constant4 : Constant  Value=eye(3)  VectorParams1D=off
  Constant5 : Constant  Value=eye(3)  VectorParams1D=off
  Constant6 : Constant  Value=G_xy  VectorParams1D=off
  Demux : Demux  Outputs=3
  Integrator : Integrator
  Matrix Multiply{1..6} (6 alike) : Product  Multiplication=Matrix(*)
  Scope : Scope
  Sum : Sum  Inputs=++++
  Sum1 : Sum  Inputs=+-|
  Terminator : Terminator
  Terminator1 : Terminator
  e_y : Outport
  v : Outport  Port=2
  wires:
  Constant2/1 -> Matrix Multiply2/1
  v_wN_hat/1 -> Scope/1, Matrix Multiply2/2
  zeta/1 -> Matrix Multiply3/2
  Constant3/1 -> Matrix Multiply3/1
  Constant1/1 -> Matrix Multiply1/1
  Matrix Multiply1/1 -> Sum/1
  Matrix Multiply3/1 -> Sum/2
  Sum/1 -> Integrator/1  "Xy_hat_dot"
  Sum1/1 -> Matrix Multiply6/2, e_y/1  "e_y"
  Constant4/1 -> Matrix Multiply4/1
  Constant5/1 -> Matrix Multiply5/1
  Matrix Multiply5/1 -> Demux/1, Sum1/2  "y_hat"
  Matrix Multiply4/1 -> Sum1/1  "y"
  Integrator/1 -> Matrix Multiply5/2, Matrix Multiply1/2  "x_hat"
  x_y/1 -> Matrix Multiply4/2
  Constant6/1 -> Matrix Multiply6/1
  Matrix Multiply6/1 -> Sum/4
  Matrix Multiply2/1 -> Sum/3
  Demux/1 -> v/1
  Demux/2 -> Terminator/1
  Demux/3 -> Terminator1/1

== system sim_finale_1/Razzo/Gravità ==
  m : Inport
  g : Inport  Port=2
  Divide : Product  Inputs=**
  Gain : Gain  Gain=-1
  Ground : Ground
  Ground1 : Ground
  Matrix Multiply1 : Product  Multiplication=Matrix(*)
  Mux : Mux  Inputs=3
  Scope : Scope
  P : Outport
  wires:
  [R_EB] -> Matrix Multiply1/1
  Divide/1 -> P/1
  m/1 -> Divide/2
  Mux/1 -> Matrix Multiply1/2
  Matrix Multiply1/1 -> Divide/1
  Ground/1 -> Mux/2
  Ground1/1 -> Mux/3
  g/1 -> Scope/1, Gain/1
  Gain/1 -> Mux/1

== system sim_finale_1/Razzo/Motore ==
  T : Inport
  TVC angles : Inport  Port=2
  Constant : Constant  Value=r_nozzle_cm
  Cross Product : matrix_library/Cross Product
  Ground2 : Ground
  Ground3 : Ground
  MATLAB Function : MATLAB Function  TreatAsAtomicUnit=on
  Matrix Multiply1 : Product  Multiplication=Matrix(*)
  Mux1 : Mux  Inputs=3
  Scope : Scope
  Scope1 : Scope
  F : Outport
  M : Outport  Port=2
  wires:
  TVC angles/1 -> MATLAB Function/1(TVC_angles)
  MATLAB Function/1(R_BN) -> Matrix Multiply1/1
  T/1 -> Mux1/1
  Ground2/1 -> Mux1/2
  Ground3/1 -> Mux1/3
  Mux1/1 -> Matrix Multiply1/2
  Matrix Multiply1/1 -> Scope/1, Cross Product/2, F/1
  Cross Product/1 -> Scope1/1, M/1
  Constant/1 -> Cross Product/1

== system sim_finale_1/Razzo/RCS attuatore ==
  rcs : Inport
  Ground : Ground
  Ground1 : Ground
  Mux : Mux  Inputs=3
  Scope : Scope
  M_rcs : Outport
  wires:
  rcs/1 -> Mux/1
  Ground/1 -> Mux/2
  Ground1/1 -> Mux/3
  Mux/1 -> Scope/1, M_rcs/1

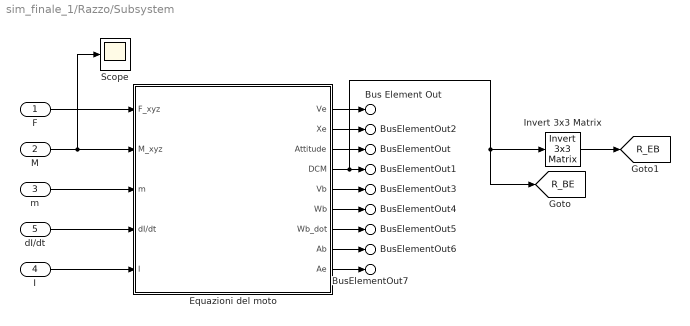
== system sim_finale_1/Razzo/Subsystem ==
  F : Inport
  M : Inport  Port=2
  m : Inport  Port=3
  I : Inport  Port=4
  dI/dt : Inport  Port=5
  Equazioni del moto : Subsystem  Variant=on
  Invert 3x3 Matrix : aerolibutil/Invert  3x3 Matrix
  Scope : Scope
  Bus Element Out : Outport  PortName=State  Element=Ve
  BusElementOut2 : Outport  PortName=State  Element=Xe
  BusElementOut : Outport  PortName=State  Element=Attitude
  BusElementOut1 : Outport  PortName=State  Element=DCM
  BusElementOut3 : Outport  PortName=State  Element=Vb
  BusElementOut4 : Outport  PortName=State  Element=Wb
  BusElementOut5 : Outport  PortName=State  Element=Wb_dot
  BusElementOut6 : Outport  PortName=State  Element=Ab
  BusElementOut7 : Outport  PortName=State  Element=Ae
  tag scope: R_BE=global, R_EB=global
  wires:
  Equazioni del moto/8(Ab) -> BusElementOut6/1
  Equazioni del moto/1(Ve) -> Bus Element Out/1
  I/1 -> Equazioni del moto/5(I)
  Equazioni del moto/2(Xe) -> BusElementOut2/1
  Equazioni del moto/9(Ae) -> BusElementOut7/1
  Equazioni del moto/3(Attitude) -> BusElementOut/1
  m/1 -> Equazioni del moto/3(m)
  M/1 -> Scope/1, Equazioni del moto/2(M_xyz)
  Equazioni del moto/5(Vb) -> BusElementOut3/1
  Equazioni del moto/7(Wb_dot) -> BusElementOut5/1
  Equazioni del moto/6(Wb) -> BusElementOut4/1
  F/1 -> Equazioni del moto/1(F_xyz)
  dI/dt/1 -> Equazioni del moto/4(dI/dt)
  Equazioni del moto/4(DCM) -> [R_BE], Invert 3x3 Matrix/1, BusElementOut1/1
  Invert 3x3 Matrix/1 -> [R_EB]

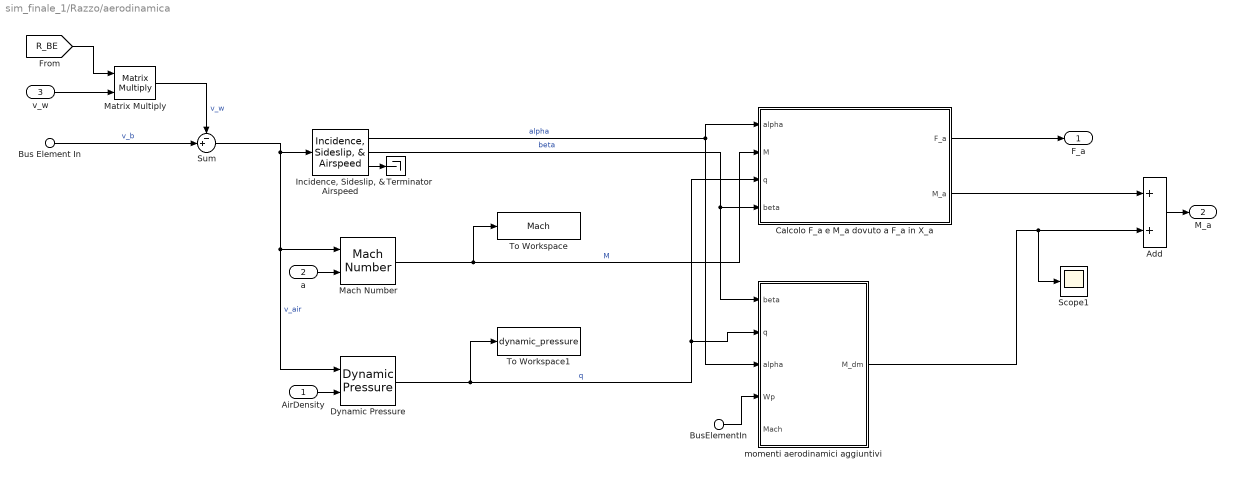
== system sim_finale_1/Razzo/aerodinamica ==
  AirDensity : Inport
  " a" : Inport  Port=2
  v_w : Inport  Port=3
  Bus Element In : Inport  Port=4  PortName=State  Element=Vb
  BusElementIn : Inport  Port=4  PortName=State  Element=Wb
  Add : Sum
  Calcolo F_a e M_a dovuto a F_a in X_a : Subsystem
  Dynamic Pressure : aerolibasang/Dynamic Pressure
  "Incidence, Sideslip, & Airspeed" : aerolibasang/Incidence, Sideslip, & Airspeed
  Mach Number : aerolibasang/Mach Number
  Matrix Multiply : Product  Multiplication=Matrix(*)
  Scope1 : Scope
  Sum : Sum  Inputs=-+|
  Terminator : Terminator
  To Workspace : ToWorkspace  VariableName=Mach  SaveFormat=Timeseries  SampleTime=-1
  To Workspace1 : ToWorkspace  VariableName=dynamic_pressure  SaveFormat=Timeseries  SampleTime=-1
  momenti aerodinamici aggiuntivi : Subsystem
  F_a : Outport
  M_a : Outport  Port=2
  wires:
  "Incidence, Sideslip, & Airspeed"/2 -> Calcolo F_a e M_a dovuto a F_a in X_a/4(beta), momenti aerodinamici aggiuntivi/1(beta)  "beta"
  AirDensity/1 -> Dynamic Pressure/2
  " a"/1 -> Mach Number/2
  "Incidence, Sideslip, & Airspeed"/1 -> Calcolo F_a e M_a dovuto a F_a in X_a/1(alpha), momenti aerodinamici aggiuntivi/3(alpha)  "alpha"
  Mach Number/1 -> To Workspace/1, Calcolo F_a e M_a dovuto a F_a in X_a/2(M)  "M"
  Add/1 -> M_a/1
  Calcolo F_a e M_a dovuto a F_a in X_a/2(M_a) -> Add/1
  Calcolo F_a e M_a dovuto a F_a in X_a/1(F_a) -> F_a/1
  BusElementIn/1 -> momenti aerodinamici aggiuntivi/4(Wp)
  Sum/1 -> "Incidence, Sideslip, & Airspeed"/1, Mach Number/1, Dynamic Pressure/1  "v_air"
  Matrix Multiply/1 -> Sum/1  "v_w"
  v_w/1 -> Matrix Multiply/2
  [R_BE] -> Matrix Multiply/1
  Bus Element In/1 -> Sum/2  "v_b"
  momenti aerodinamici aggiuntivi/1(M_dm) -> Scope1/1, Add/2
  "Incidence, Sideslip, & Airspeed"/3 -> Terminator/1
  Dynamic Pressure/1 -> To Workspace1/1, Calcolo F_a e M_a dovuto a F_a in X_a/3(q), momenti aerodinamici aggiuntivi/2(q)  "q"

== system sim_finale_1/Razzo/massa ==
  T : Inport
  massa costante : Subsystem  VariantControl=massa_variabile==false
  massa variabile : Subsystem  VariantControl=massa_variabile==true
  I : Outport
  I_dot : Outport  Port=2
  m : Outport  Port=3

== system sim_finale_1/Variant Subsystem/meno reale ==
  State : Inport
  Ambiente : Subsystem
  Env : Outport
  wires:
  Ambiente/1(Environment) -> Env/1
  State/1 -> Ambiente/1(State)

== system sim_finale_1/Variant Subsystem/reale ==
  State : Inport
  Ambiente1 : Subsystem
  Env : Outport
  tag scope: Env=global
  wires:
  Ambiente1/1(Environment) -> Env/1, [Env]
  State/1 -> Ambiente1/1(State)

== system sim_finale_1/Controllore/Variant Subsystem/Controllore 2: rlocus sforzo di TVC minore  ==
  Attitude : Inport
  Demux1 : Demux  Outputs=3
  LTI System : cstblocks/LTI System  sys=G_6_y  IC=[]  PadeOrder=0
  LTI System1 : cstblocks/LTI System  sys=G_6_y  IC=[]  PadeOrder=0
  Mux1 : Mux  Inputs=2
  Terminator : Terminator
  TVC angles : Outport
  wires:
  Demux1/1 -> Terminator/1
  LTI System1/1 -> Mux1/2  "eta"
  Mux1/1 -> TVC angles/1
  LTI System/1 -> Mux1/1  "zeta"
  Attitude/1 -> Demux1/1
  Demux1/2 -> LTI System1/1  "theta"
  Demux1/3 -> LTI System/1  "psi"

== system sim_finale_1/Controllore/Variant Subsystem/PID ==
  Attitude : Inport
  Demux1 : Demux  Outputs=3
  LTI System : cstblocks/LTI System  sys=PID_y  IC=[]  PadeOrder=0
  LTI System1 : cstblocks/LTI System  sys=PID_p  IC=[]  PadeOrder=0
  Mux1 : Mux  Inputs=2
  Terminator : Terminator
  TVC angles : Outport
  wires:
  LTI System/1 -> Mux1/1  "zeta"
  Demux1/3 -> LTI System/1  "psi"
  Demux1/1 -> Terminator/1
  Mux1/1 -> TVC angles/1
  LTI System1/1 -> Mux1/2  "eta"
  Demux1/2 -> LTI System1/1  "theta"
  Attitude/1 -> Demux1/1

== system sim_finale_1/Controllore/Variant Subsystem/tune ==
  Attitude : Inport
  Demux1 : Demux  Outputs=3
  Mux1 : Mux  Inputs=2
  PID Controller : slpidlib/PID Controller  Controller=PID  Form=Parallel  TimeDomain=Continuous-time  UseExternalTs=off  SampleTime=-1  IntegratorMethod=Forward Euler  FilterMethod=Forward Euler  ControllerParametersSource=internal  P=1  I=1  UseKiTs=off  D=0  UseExternalDerivativeSource=off  N=100  UseFilter=on  TunerSelectOption=Transfer Function Based (PID Tuner App)  InitialConditionSource=internal  InitialConditionForIntegrator=0  InitialConditionForFilter=0  DifferentiatorICPrevScaledInput=0  ExternalReset=none  TrackingMode=off  Kt=1  LimitOutput=off  SatLimitsSource=internal  UpperSaturationLimit=inf  LowerSaturationLimit=-inf  LinearizeAsGain=on  AntiWindupMode=none  Kb=1  LimitIntegrator=off  UpperIntegratorSaturationLimit=inf  LowerIntegratorSaturationLimit=-inf  POutMin=[]  POutMax=[]  IOutMin=[]  IOutMax=[]  DOutMin=[]  DOutMax=[]  NOutMin=[]  NOutMax=[]  SumOutMin=[]  SumOutMax=[]  SaturationOutMin=[]  SaturationOutMax=[]  PParamMin=[]  PParamMax=[]  IParamMin=[]  IParamMax=[]  DParamMin=[]  DParamMax=[]  NParamMin=[]  NParamMax=[]  KbParamMin=[]  KbParamMax=[]  KtParamMin=[]  KtParamMax=[]  KbOutMin=[]  KbOutMax=[]  KtOutMin=[]  KtOutMax=[]  IntegratorOutMin=[]  IntegratorOutMax=[]  FilterOutMin=[]  FilterOutMax=[]  SumI1OutMin=[]  SumI1OutMax=[]  SumI2OutMin=[]  SumI2OutMax=[]  SumI3OutMin=[]  SumI3OutMax=[]  SumI4OutMin=[]  SumI4OutMax=[]  SumDOutMin=[]  SumDOutMax=[]  DifferentiatorOutMin=[]  DifferentiatorOutMax=[]  FilterDiffOutCoefMin=[]  FilterDiffOutCoefMax=[]  ReciprocalOutMin=[]  ReciprocalOutMax=[]  SumDenOutMin=[]  SumDenOutMax=[]  SumNumOutMin=[]  SumNumOutMax=[]  DivideOutMin=[]  DivideOutMax=[]  UdiffTsProdOutMin=[]  UdiffTsProdOutMax=[]  NTsProdOutMin=[]  NTsProdOutMax=[]  UintegralTsProdOutMin=[]  UintegralTsProdOutMax=[]  UngainTsProdOutMin=[]  UngainTsProdOutMax=[]  ClampingZeroOutDataTypeStr=Inherit: Inherit via back propagation  ClampingZeroOutMin=[]  ClampingZeroOutMax=[]  FilterDenConstantOutDataTypeStr=Inherit: Inherit via back propagation  FilterDenConstantOutMin=[]  FilterDenConstantOutMax=[]  PCopyOutDataTypeStr=Inherit: Inherit via back propagation  PCopyOutMin=[]  PCopyOutMax=[]  NCopyOutDataTypeStr=Inherit: Inherit via back propagation  NCopyOutMin=[]  NCopyOutMax=[]  IntegratorContinuousStateAttributes=''  IntegratorStateMustResolveToSignalObject=off  IntegratorRTWStateStorageClass=Auto  FilterContinuousStateAttributes=''  FilterStateMustResolveToSignalObject=off  FilterRTWStateStorageClass=Auto  ParallelPVariant=InternalParameters  IdealPVariant=Disabled  IVariant=InternalParameters  DVariant=InternalParameters  IntegratorVariant=Continuous  SatVariant=Disabled  AWVariant=Passthrough  PCopyVariant=Disabled  TRVariant=Disabled  FdbkBlocksVariant=Forward  IdealPFdbkVariant=Disabled  SatFdbkVariant=Disabled  DerivativeFilterVariant=ContFilter  NVariant=InternalParameters  NCopyVariant=Disabled  FilterICVariant=InternalICsFilter  IntegratorICVariant=InternalICs  ExternalResetVariant=Disabled  TRSumVariant=Passthrough  SumFdbkVariant=Disabled  SumVariant=Sum_PID  TsampFilterVariant=InternalTs  TsampNgainVariant=Passthrough  TsampIntegralVariant=Disabled_SignalSpec  ExternalSaturationOutDataTypeStr=Inherit: Same as second input  DerivativeSourceVariant=ErrorSignal
  PID Controller1 : slpidlib/PID Controller  Controller=PID  Form=Parallel  TimeDomain=Continuous-time  UseExternalTs=off  SampleTime=-1  IntegratorMethod=Forward Euler  FilterMethod=Forward Euler  ControllerParametersSource=internal  P=1  I=1  UseKiTs=off  D=0  UseExternalDerivativeSource=off  N=100  UseFilter=on  TunerSelectOption=Transfer Function Based (PID Tuner App)  InitialConditionSource=internal  InitialConditionForIntegrator=0  InitialConditionForFilter=0  DifferentiatorICPrevScaledInput=0  ExternalReset=none  TrackingMode=off  Kt=1  LimitOutput=off  SatLimitsSource=internal  UpperSaturationLimit=inf  LowerSaturationLimit=-inf  LinearizeAsGain=on  AntiWindupMode=none  Kb=1  LimitIntegrator=off  UpperIntegratorSaturationLimit=inf  LowerIntegratorSaturationLimit=-inf  POutMin=[]  POutMax=[]  IOutMin=[]  IOutMax=[]  DOutMin=[]  DOutMax=[]  NOutMin=[]  NOutMax=[]  SumOutMin=[]  SumOutMax=[]  SaturationOutMin=[]  SaturationOutMax=[]  PParamMin=[]  PParamMax=[]  IParamMin=[]  IParamMax=[]  DParamMin=[]  DParamMax=[]  NParamMin=[]  NParamMax=[]  KbParamMin=[]  KbParamMax=[]  KtParamMin=[]  KtParamMax=[]  KbOutMin=[]  KbOutMax=[]  KtOutMin=[]  KtOutMax=[]  IntegratorOutMin=[]  IntegratorOutMax=[]  FilterOutMin=[]  FilterOutMax=[]  SumI1OutMin=[]  SumI1OutMax=[]  SumI2OutMin=[]  SumI2OutMax=[]  SumI3OutMin=[]  SumI3OutMax=[]  SumI4OutMin=[]  SumI4OutMax=[]  SumDOutMin=[]  SumDOutMax=[]  DifferentiatorOutMin=[]  DifferentiatorOutMax=[]  FilterDiffOutCoefMin=[]  FilterDiffOutCoefMax=[]  ReciprocalOutMin=[]  ReciprocalOutMax=[]  SumDenOutMin=[]  SumDenOutMax=[]  SumNumOutMin=[]  SumNumOutMax=[]  DivideOutMin=[]  DivideOutMax=[]  UdiffTsProdOutMin=[]  UdiffTsProdOutMax=[]  NTsProdOutMin=[]  NTsProdOutMax=[]  UintegralTsProdOutMin=[]  UintegralTsProdOutMax=[]  UngainTsProdOutMin=[]  UngainTsProdOutMax=[]  ClampingZeroOutDataTypeStr=Inherit: Inherit via back propagation  ClampingZeroOutMin=[]  ClampingZeroOutMax=[]  FilterDenConstantOutDataTypeStr=Inherit: Inherit via back propagation  FilterDenConstantOutMin=[]  FilterDenConstantOutMax=[]  PCopyOutDataTypeStr=Inherit: Inherit via back propagation  PCopyOutMin=[]  PCopyOutMax=[]  NCopyOutDataTypeStr=Inherit: Inherit via back propagation  NCopyOutMin=[]  NCopyOutMax=[]  IntegratorContinuousStateAttributes=''  IntegratorStateMustResolveToSignalObject=off  IntegratorRTWStateStorageClass=Auto  FilterContinuousStateAttributes=''  FilterStateMustResolveToSignalObject=off  FilterRTWStateStorageClass=Auto  ParallelPVariant=InternalParameters  IdealPVariant=Disabled  IVariant=InternalParameters  DVariant=InternalParameters  IntegratorVariant=Continuous  SatVariant=Disabled  AWVariant=Passthrough  PCopyVariant=Disabled  TRVariant=Disabled  FdbkBlocksVariant=Forward  IdealPFdbkVariant=Disabled  SatFdbkVariant=Disabled  DerivativeFilterVariant=ContFilter  NVariant=InternalParameters  NCopyVariant=Disabled  FilterICVariant=InternalICsFilter  IntegratorICVariant=InternalICs  ExternalResetVariant=Disabled  TRSumVariant=Passthrough  SumFdbkVariant=Disabled  SumVariant=Sum_PID  TsampFilterVariant=InternalTs  TsampNgainVariant=Passthrough  TsampIntegralVariant=Disabled_SignalSpec  ExternalSaturationOutDataTypeStr=Inherit: Same as second input  DerivativeSourceVariant=ErrorSignal
  Terminator : Terminator
  TVC angles : Outport
  wires:
  PID Controller/1 -> Mux1/1  "zeta"
  Demux1/3 -> PID Controller/1  "psi"
  Demux1/1 -> Terminator/1
  Mux1/1 -> TVC angles/1
  PID Controller1/1 -> Mux1/2  "eta"
  Demux1/2 -> PID Controller1/1  "theta"
  Attitude/1 -> Demux1/1

== system sim_finale_1/Controllore/Variant Subsystem1/No controllore velocità ==
  V_b : Inport
  Constant : Constant  Value=Attitude_riferimento
  Terminator : Terminator
  Out1 : Outport
  wires:
  V_b/1 -> Terminator/1
  Constant/1 -> Out1/1

== system sim_finale_1/Controllore/Variant Subsystem1/PID ==
  V_b : Inport
  Demux : Demux  Outputs=3
  Ground : Ground
  LTI System : cstblocks/LTI System  sys=G_7_p  IC=[]  PadeOrder=0
  LTI System1 : cstblocks/LTI System  sys=G_7_y  IC=[]  PadeOrder=0
  Mux : Mux  Inputs=3
  Terminator : Terminator
  Out1 : Outport
  wires:
  V_b/1 -> Demux/1
  Mux/1 -> Out1/1
  Demux/1 -> Terminator/1
  Ground/1 -> Mux/1
  Demux/2 -> LTI System/1
  Demux/3 -> LTI System1/1
  LTI System/1 -> Mux/2
  LTI System1/1 -> Mux/3

== system sim_finale_1/Controllore/Variant Subsystem2/mio controllo ==
  Attitude : Inport
  Demux2 : Demux  Outputs=3
  LTI System : cstblocks/LTI System  sys=G_roll  IC=[]  PadeOrder=0
  Terminator : Terminator
  Terminator1 : Terminator
  RCS : Outport
  wires:
  Demux2/1 -> LTI System/1  "chi"
  Attitude/1 -> Demux2/1
  Demux2/3 -> Terminator1/1  "psi"
  Demux2/2 -> Terminator/1  "theta"
  LTI System/1 -> RCS/1

== system sim_finale_1/Controllore/Variant Subsystem2/sbagliato ==
  Attitude : Inport
  Demux2 : Demux  Outputs=3
  LTI System : cstblocks/LTI System  sys=G_roll_sba  IC=[]  PadeOrder=0
  Terminator : Terminator
  Terminator1 : Terminator
  RCS : Outport
  wires:
  Demux2/1 -> LTI System/1  "chi"
  Attitude/1 -> Demux2/1
  Demux2/3 -> Terminator1/1  "psi"
  Demux2/2 -> Terminator/1  "theta"
  LTI System/1 -> RCS/1

== system sim_finale_1/Controllore/Variant Subsystem2/tune ==
  Attitude : Inport
  Demux2 : Demux  Outputs=3
  PID Controller1 : slpidlib/PID Controller  Controller=PID  Form=Parallel  TimeDomain=Continuous-time  UseExternalTs=off  SampleTime=-1  IntegratorMethod=Forward Euler  FilterMethod=Forward Euler  ControllerParametersSource=internal  P=264600.900282427  I=44368.5448911241  UseKiTs=off  D=382704.214968411  UseExternalDerivativeSource=off  N=17.2469682941307  UseFilter=on  TunerSelectOption=Transfer Function Based (PID Tuner App)  InitialConditionSource=internal  InitialConditionForIntegrator=0  InitialConditionForFilter=0  DifferentiatorICPrevScaledInput=0  ExternalReset=none  TrackingMode=off  Kt=1  LimitOutput=off  SatLimitsSource=internal  UpperSaturationLimit=inf  LowerSaturationLimit=-inf  LinearizeAsGain=on  AntiWindupMode=none  Kb=1  LimitIntegrator=off  UpperIntegratorSaturationLimit=inf  LowerIntegratorSaturationLimit=-inf  POutMin=[]  POutMax=[]  IOutMin=[]  IOutMax=[]  DOutMin=[]  DOutMax=[]  NOutMin=[]  NOutMax=[]  SumOutMin=[]  SumOutMax=[]  SaturationOutMin=[]  SaturationOutMax=[]  PParamMin=[]  PParamMax=[]  IParamMin=[]  IParamMax=[]  DParamMin=[]  DParamMax=[]  NParamMin=[]  NParamMax=[]  KbParamMin=[]  KbParamMax=[]  KtParamMin=[]  KtParamMax=[]  KbOutMin=[]  KbOutMax=[]  KtOutMin=[]  KtOutMax=[]  IntegratorOutMin=[]  IntegratorOutMax=[]  FilterOutMin=[]  FilterOutMax=[]  SumI1OutMin=[]  SumI1OutMax=[]  SumI2OutMin=[]  SumI2OutMax=[]  SumI3OutMin=[]  SumI3OutMax=[]  SumI4OutMin=[]  SumI4OutMax=[]  SumDOutMin=[]  SumDOutMax=[]  DifferentiatorOutMin=[]  DifferentiatorOutMax=[]  FilterDiffOutCoefMin=[]  FilterDiffOutCoefMax=[]  ReciprocalOutMin=[]  ReciprocalOutMax=[]  SumDenOutMin=[]  SumDenOutMax=[]  SumNumOutMin=[]  SumNumOutMax=[]  DivideOutMin=[]  DivideOutMax=[]  UdiffTsProdOutMin=[]  UdiffTsProdOutMax=[]  NTsProdOutMin=[]  NTsProdOutMax=[]  UintegralTsProdOutMin=[]  UintegralTsProdOutMax=[]  UngainTsProdOutMin=[]  UngainTsProdOutMax=[]  ClampingZeroOutDataTypeStr=Inherit: Inherit via back propagation  ClampingZeroOutMin=[]  ClampingZeroOutMax=[]  FilterDenConstantOutDataTypeStr=Inherit: Inherit via back propagation  FilterDenConstantOutMin=[]  FilterDenConstantOutMax=[]  PCopyOutDataTypeStr=Inherit: Inherit via back propagation  PCopyOutMin=[]  PCopyOutMax=[]  NCopyOutDataTypeStr=Inherit: Inherit via back propagation  NCopyOutMin=[]  NCopyOutMax=[]  IntegratorContinuousStateAttributes=''  IntegratorStateMustResolveToSignalObject=off  IntegratorRTWStateStorageClass=Auto  FilterContinuousStateAttributes=''  FilterStateMustResolveToSignalObject=off  FilterRTWStateStorageClass=Auto  ParallelPVariant=InternalParameters  IdealPVariant=Disabled  IVariant=InternalParameters  DVariant=InternalParameters  IntegratorVariant=Continuous  SatVariant=Disabled  AWVariant=Passthrough  PCopyVariant=Disabled  TRVariant=Disabled  FdbkBlocksVariant=Forward  IdealPFdbkVariant=Disabled  SatFdbkVariant=Disabled  DerivativeFilterVariant=ContFilter  NVariant=InternalParameters  NCopyVariant=Disabled  FilterICVariant=InternalICsFilter  IntegratorICVariant=InternalICs  ExternalResetVariant=Disabled  TRSumVariant=Passthrough  SumFdbkVariant=Disabled  SumVariant=Sum_PID  TsampFilterVariant=InternalTs  TsampNgainVariant=Passthrough  TsampIntegralVariant=Disabled_SignalSpec  ExternalSaturationOutDataTypeStr=Inherit: Same as second input  DerivativeSourceVariant=ErrorSignal
  Terminator : Terminator
  Terminator1 : Terminator
  RCS : Outport
  wires:
  Demux2/2 -> Terminator/1  "theta"
  Demux2/3 -> Terminator1/1  "psi"
  Attitude/1 -> Demux2/1
  Demux2/1 -> PID Controller1/1  "chi"
  PID Controller1/1 -> RCS/1

== system sim_finale_1/Controllore/reiezione del disturbo/Vuoto ==
  v_wE_hat : Inport
  v_wN_hat : Inport  Port=2
  TVC_angles_z_rejection : Outport

== system sim_finale_1/Controllore/reiezione del disturbo/frequenza controllore 3 ==
  v_wE_hat : Inport
  v_wN_hat : Inport  Port=2
  LTI System : cstblocks/LTI System  sys=K_3_y  IC=[]  PadeOrder=0
  LTI System1 : cstblocks/LTI System  sys=K_3_p  IC=[]  PadeOrder=0
  Mux : Mux  Inputs=2
  TVC_angles_z_rejection : Outport
  wires:
  v_wE_hat/1 -> LTI System1/1
  Mux/1 -> TVC_angles_z_rejection/1
  LTI System/1 -> Mux/1  "zeta"
  v_wN_hat/1 -> LTI System/1
  LTI System1/1 -> Mux/2  "zeta"

== system sim_finale_1/Controllore/reiezione del disturbo/frequenza controllore 4 ==
  v_wE_hat : Inport
  v_wN_hat : Inport  Port=2
  LTI System : cstblocks/LTI System  sys=K_4_y  IC=[]  PadeOrder=0
  LTI System1 : cstblocks/LTI System  sys=K_4_p  IC=[]  PadeOrder=0
  Mux : Mux  Inputs=2
  TVC_angles_z_rejection : Outport
  wires:
  Mux/1 -> TVC_angles_z_rejection/1
  LTI System/1 -> Mux/1  "zeta"
  v_wN_hat/1 -> LTI System/1
  v_wE_hat/1 -> LTI System1/1
  LTI System1/1 -> Mux/2  "etha"

== system sim_finale_1/Controllore/reiezione del disturbo/frequenza controllore 7 ==
  v_wE_hat : Inport
  v_wN_hat : Inport  Port=2
  LTI System : cstblocks/LTI System  sys=K_7_y  IC=[]  PadeOrder=0
  LTI System1 : cstblocks/LTI System  sys=K_7_p  IC=[]  PadeOrder=0
  Mux : Mux  Inputs=2
  TVC_angles_z_rejection : Outport
  wires:
  Mux/1 -> TVC_angles_z_rejection/1
  LTI System/1 -> Mux/1  "zeta"
  v_wN_hat/1 -> LTI System/1
  v_wE_hat/1 -> LTI System1/1
  LTI System1/1 -> Mux/2  "etha"

== system sim_finale_1/Razzo/Subsystem/Equazioni del moto ==
  F_xyz : Inport
  M_xyz : Inport  Port=2
  m : Inport  Port=3
  dI/dt : Inport  Port=4
  I : Inport  Port=5
  Eq. massa costante : Subsystem  VariantControl=massa_variabile==false
  Eq. massa variabile : Subsystem  VariantControl=massa_variabile==true
  Ve : Outport
  Xe : Outport  Port=2
  Attitude : Outport  Port=3
  DCM : Outport  Port=4
  Vb : Outport  Port=5
  Wb : Outport  Port=6
  Wb_dot : Outport  Port=7
  Ab : Outport  Port=8
  Ae : Outport  Port=9

== system sim_finale_1/Razzo/aerodinamica/Calcolo F_a e M_a dovuto a F_a in X_a ==
  alpha : Inport
  M : Inport  Port=2
  q : Inport  Port=3
  beta : Inport  Port=4
  C_A C_N_alpha : Subsystem  Variant=on
  Constant : Constant  Value=S_rif
  Constant1 : Constant  Value=r_cp_cm
  Cross Product : matrix_library/Cross Product
  Gain : Gain  Gain=-1
  Mux1 : Mux  Inputs=3
  Product2 : Product
  Product3 : Product
  Product4 : Product  Inputs=3
  Scope : Scope
  Scope1 : Scope
  To Workspace1 : ToWorkspace  VariableName=C_A_table  SaveFormat=Timeseries  SampleTime=-1
  To Workspace2 : ToWorkspace  VariableName=C_N_alpha_table  SaveFormat=Timeseries  SampleTime=-1
  F_a : Outport
  M_a : Outport  Port=2
  wires:
  q/1 -> Product4/1
  Constant/1 -> Product4/2
  Gain/1 -> F_a/1, Cross Product/2
  Cross Product/1 -> M_a/1
  Constant1/1 -> Cross Product/1
  Product2/1 -> Mux1/2
  Product3/1 -> Mux1/3
  Mux1/1 -> Product4/3
  M/1 -> C_A C_N_alpha/1(Mach)
  Product4/1 -> Gain/1
  C_A C_N_alpha/1(C_A) -> To Workspace1/1, Mux1/1, Scope/1  "C_A"
  alpha/1 -> Product3/2
  beta/1 -> Product2/2
  C_A C_N_alpha/2(C_N_alpha) -> Scope1/1, To Workspace2/1, Product3/1, Product2/1  "C_N_alpha"
